simulink model "pendulum1"  (R2021b)
settings: Solver=FixedStepAuto  StartTime=0.0  StopTime=10  FixedStep=0.01  RelTol=1e-3
libraries: cstblocks x1
settings Model: Creator=DELL  LastModifiedBy=DELL

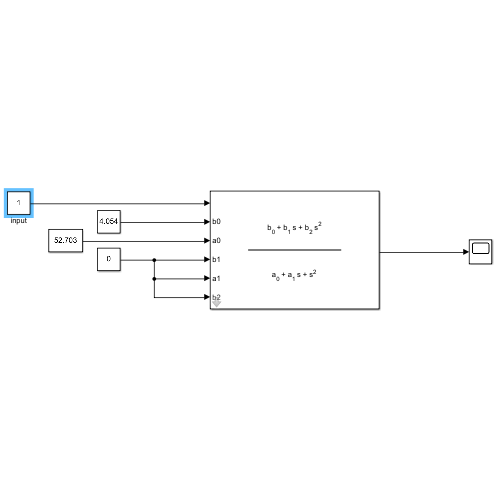
[thumbnail: Simulink's stored preview of the top-level diagram]
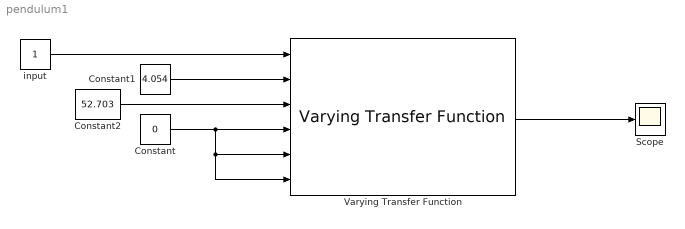
== system pendulum1 ==
  Constant : Constant  Value=0
  Constant1 : Constant  Value=4.054
  Constant2 : Constant  Value=52.703
  Scope : Scope
  Varying Transfer Function : cstblocks/Linear Parameter Varying/Varying Transfer Function  N=2
  input : Constant
  wires:
  Constant/1 -> Varying Transfer Function/6, Varying Transfer Function/5, Varying Transfer Function/4
  Varying Transfer Function/1 -> Scope/1
  input/1 -> Varying Transfer Function/1
  Constant1/1 -> Varying Transfer Function/2
  Constant2/1 -> Varying Transfer Function/3
